simulink library "resettableTimer"  (R2018a)
settings: Solver=VariableStepAuto  StartTime=0.0  StopTime=10.0  RelTol=1e-3
libraries: dspsigops x1
settings Model: Creator=mitch  LastModifiedBy=mitch

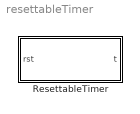
== system resettableTimer ==
  ResettableTimer : Subsystem

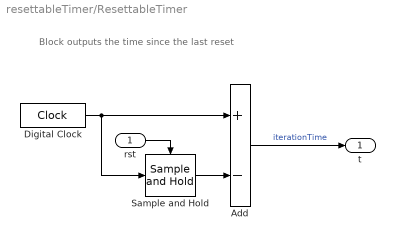
== system resettableTimer/ResettableTimer ==
  note: Block outputs the time since the last reset
  rst : Inport  OutDataTypeStr=boolean
  Add : Sum  Inputs=+-
  Digital Clock : DigitalClock  SampleTime=sm.Ts
  Sample and Hold : dspsigops/Sample and Hold  trig=Rising edge  initCond=0  latchinput=off
  t : Outport
  wires:
  Add/1 -> t/1  "iterationTime"
  Sample and Hold/1 -> Add/2
  rst/1 -> Sample and Hold/Trigger
  Digital Clock/1 -> Sample and Hold/1, Add/1
